simulink model "Quadruped2D_Simulink"  (R2023b)
settings: Solver=VariableStepAuto  StartTime=0.0  StopTime=T  RelTol=1e-3
undefined symbols (not defined in the file): control, dt, Kd, option, pFootRi, Q_TO, robotParams, robotStruct, X, Y, Z
libraries: sm_lib x185, nesl_utility x44
(part 5 of 5)

== matlab function Quadruped2D_Simulink/MATLAB Function1 ==
  data: t input; T_FL output; Q input; tau input; dt_sim input; q input; dq input; T_FR output; T_RL output; T_RR output
function [T_FL, T_FR, T_RL, T_RR] = jointPD_Quad2D(t, Q, tau, dt_sim, q, dq)

Kp = 100;
Kd = 1;

KpHip = 300;
KdHip = 3;
N_input = length(tau(1,:));

%find index of nearest TO timestep
k = round(t/dt_sim)+1;

%upper bound of index is max length of simulation
k = min(k,N_input);

%%
t_active = 0;
%if prior to simulation start, zero out torques
if t <= t_active
    T_FL = zeros(3,1);
    T_FR = zeros(3,1);
    T_RL = zeros(3,1);
    T_RR = zeros(3,1);
    q_diff = zeros(24, 1);
    dq_diff = zeros(24, 1);
else

    tau_hip_roll_des_k = 0;
    q_hip_roll_des_k = 0;
    dq_hip_roll_des_k = 0;

    tau_hip_pitch_F_des_k = tau(1,k)/2;
    q_hip_pitch_F_des_k = Q(4,k);

    tau_knee_F_des_k = tau(2,k)/2;
    q_knee_F_des_k = Q(5,k);

    tau_hip_pitch_R_des_k = tau(3,k)/2;
    q_hip_pitch_R_des_k = Q(6,k);
    
    tau_knee_R_des_k = tau(4,k)/2;
    q_knee_R_des_k = Q(7,k);

    if k == 1 || k == N_input
        dq_hip_pitch_F_des_k = 0; 
        dq_knee_F_des_k = 0;
        dq_hip_pitch_R_des_k = 0; 
        dq_knee_R_des_k = 0;
    else
        dq_hip_pitch_F_des_k = (Q(4,k)-Q(4,k-1))/(dt_sim);  
        dq_knee_F_des_k = (Q(5,k)-Q(5,k-1))/(dt_sim); 
        dq_hip_pitch_R_des_k = (Q(6,k)-Q(6,k-1))/(dt_sim);  
        dq_knee_R_des_k = (Q(7,k)-Q(7,k-1))/(dt_sim); 
    end
    qFL = q(1:3);
    qFR = q(4:6);
    qRL = q(7:9);
    qRR = q(10:12);

    dqFL = dq(1:3);
    dqFR = dq(4:6);
    dqRL = dq(7:9);
    dqRR = dq(10:12);

    tau_hip_roll_FL = tau_hip_roll_des_k + KpHip * (q_hip_roll_des_k - qFL(1)) + KdHip * (dq_hip_roll_des_k - dqFL(1));
    tau_hip_pitch_FL = tau_hip_pitch_F_des_k + Kp * (q_hip_pitch_F_des_k - qFL(2)) + Kd * (dq_hip_pitch_F_des_k - dqFL(2));
    tau_knee_FL = tau_knee_F_des_k + Kp * (q_knee_F_des_k - qFL(3)) + Kd * (dq_knee_F_des_k - dqFL(3));

    tau_hip_roll_FR = tau_hip_roll_des_k + KpHip * (q_hip_roll_des_k - qFR(1)) + KdHip * (dq_hip_roll_des_k - dqFR(1));
    tau_hip_pitch_FR = tau_hip_pitch_F_des_k + Kp * (q_hip_pitch_F_des_k - qFR(2)) + Kd * (dq_hip_pitch_F_des_k - dqFR(2));
    tau_knee_FR = tau_knee_F_des_k + Kp * (q_knee_F_des_k - qFR(3)) + Kd * (dq_knee_F_des_k - dqFR(3));

    tau_hip_roll_RL = tau_hip_roll_des_k + KpHip * (q_hip_roll_des_k - qRL(1)) + KdHip * (dq_hip_roll_des_k - dqRL(1));
    tau_hip_pitch_RL = tau_hip_pitch_R_des_k + Kp * (q_hip_pitch_R_des_k - qRL(2)) + Kd * (dq_hip_pitch_R_des_k - dqRL(2));
    tau_knee_RL = tau_knee_R_des_k + Kp * (q_knee_R_des_k - qRL(3)) + Kd * (dq_knee_R_des_k - dqRL(3));

    tau_hip_roll_RR = tau_hip_roll_des_k + KpHip * (q_hip_roll_des_k - qRR(1)) + KdHip * (dq_hip_roll_des_k - dqRR(1));
    tau_hip_pitch_RR = tau_hip_pitch_R_des_k + Kp * (q_hip_pitch_R_des_k - qRR(2)) + Kd * (dq_hip_pitch_R_des_k - dqRR(2));
    tau_knee_RR = tau_knee_R_des_k + Kp * (q_knee_R_des_k - qRR(3)) + Kd * (dq_knee_R_des_k - dqRR(3));

    T_FL = [tau_hip_roll_FL; tau_hip_pitch_FL; tau_knee_FL];
    T_FR = [tau_hip_roll_FR; tau_hip_pitch_FR; tau_knee_FR];
    T_RL = [tau_hip_roll_RL; tau_hip_pitch_RL; tau_knee_RL];
    T_RR = [tau_hip_roll_RR; tau_hip_pitch_RR; tau_knee_RR];

    q_diffFL = [q_hip_roll_des_k; qFL(1); q_hip_pitch_F_des_k; qFL(2); q_knee_F_des_k; qFL(3)];
    q_diffFR = [q_hip_roll_des_k; qFR(1); q_hip_pitch_F_des_k; qFR(2); q_knee_F_des_k; qFR(3)];
    q_diffRL = [q_hip_roll_des_k; qRL(1); q_hip_pitch_R_des_k; qRL(2); q_knee_R_des_k; qRL(3)];
    q_diffRR = [q_hip_roll_des_k; qRR(1); q_hip_pitch_R_des_k; qRR(2); q_knee_R_des_k; qRR(3)];

    dq_diffFL = [dq_hip_roll_des_k; dqFL(1); dq_hip_pitch_F_des_k; dqFL(2); dq_knee_F_des_k; dqFL(3)];
    dq_diffFR = [dq_hip_roll_des_k; dqFR(1); dq_hip_pitch_F_des_k; dqFR(2); dq_knee_F_des_k; dqFR(3)];
    dq_diffRL = [dq_hip_roll_des_k; dqRL(1); dq_hip_pitch_R_des_k; dqRL(2); dq_knee_R_des_k; dqRL(3)];
    dq_diffRR = [dq_hip_roll_des_k; dqRR(1); dq_hip_pitch_R_des_k; dqRR(2); dq_knee_R_des_k; dqRR(3)];

    q_diff = [q_diffFL; q_diffFR; q_diffRL; q_diffRR];
    dq_diff = [dq_diffFL; dq_diffFR; dq_diffRL; dq_diffRR];
end
